simulink model "V5_Diagrama_completo_prolijo"  (R2023b)
settings: Solver=VariableStepAuto  StartTime=0.0  StopTime=15  FixedStep=0.00001  RelTol=1e-3
values from neighbouring files (symbols this model uses):
  A_corriente = [0 1; -wn_corriente^2 -2*zeta_corriente*wn_corriente]    [SensoresReales.m]
  A_inv = [0 1; -wn_inv^2 -2*zeta_inv*wn_inv]    [SensoresReales.m]
  A_temp = -1/tau_temp    (= -0.05)    [SensoresReales.m]
  A_tita = [0 1; -wn_tita^2 -2*zeta_tita*wn_tita]    [SensoresReales.m]
  B_corriente = [0; wn_corriente^2]    [SensoresReales.m]
  B_inv = [0; wn_inv^2]    [SensoresReales.m]
  B_temp = 1/tau_temp    (= 0.05)    [SensoresReales.m]
  B_tita = [0; wn_tita^2]    [SensoresReales.m]
  ba = Jeq * n * wn    [PolosPID.m]
  C_corriente = [1 0]    [SensoresReales.m]
  C_inv = [1 0]    [SensoresReales.m]
  C_temp = 1    [SensoresReales.m]
  C_tita = [1 0]    [SensoresReales.m]
  D_corriente = 0    [SensoresReales.m]
  D_inv = 0    [SensoresReales.m]
  D_temp = 0    [SensoresReales.m]
  D_tita = 0    [SensoresReales.m]
  ketita = double(sol.ketita_s)    [PIDPolosObsReducidoEst.m]    (also in PolosObsReducidoEst.m)
  kew = double(sol.kew_s)    [PIDPolosObsReducidoEst.m]    (also in PolosObsReducidoEst.m)
  kewint = double(sol.kewint_s)    [PIDPolosObsReducidoEst.m]    (also in PolosObsReducidoEst.m = 0)
  Ksa = Jeq * n * wn^2    [PolosPID.m]
  Ksia = Jeq * wn^3    [PolosPID.m]
  Ra_prima = Lq/Tau    [RaLazoControlCorriente.m]
  Vs_max = 48 * sqrt(2) / sqrt(3)    [SensoresReales.m]
undefined symbols (not defined in the file or in its folder): alfa, beq, Cts, g, id0, io0, iq0, Jeq, KEeq, kl, KTeq, lambda_m, Ld, Lls, Lq, Pp, r, Rs, Rts_amb, tita0, Ts0, wm0
libraries: simulink_extras x8, eeTransforms x4, SignalEditorBlockLib x3, simulink x3
settings Model: Creator=Julian  LastModifiedBy=Julian

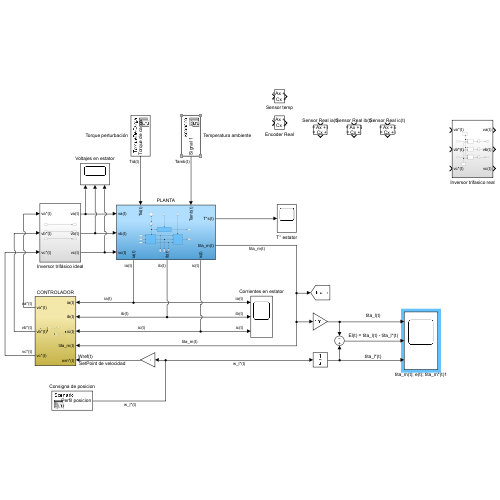
[thumbnail: Simulink's stored preview of the top-level diagram]
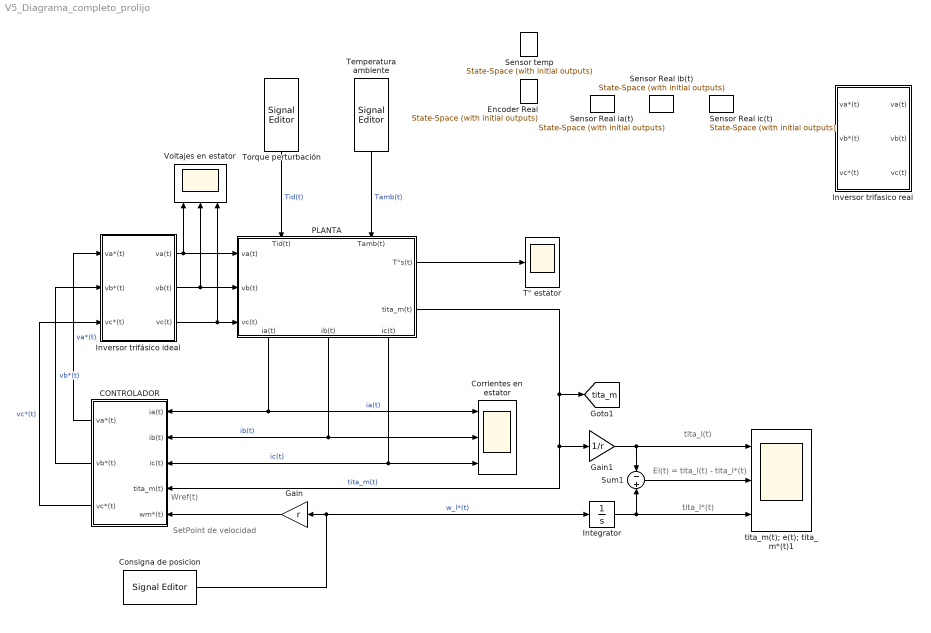
== system V5_Diagrama_completo_prolijo ==
  note: Wref(t)
  note: El(t) = tita_l(t) - tita_l*(t)
  note: tita_l*(t)
  note: tita_l(t)
  note: SetPoint de velocidad
  CONTROLADOR : Subsystem
  Consigna de posicion : SignalEditorBlockLib/Signal Editor  FileName=C:\Users\Julian\OneDrive\Documentos\UNC\Cuarto\AyME\Proyecto\Simulink\Señales\PerfilTrapezoidalVelocidadMejorado.mat  ActiveScenario=Scenario  ActiveSignal=Perfil posicion  IsBus=off  OutputBusObjectStr=Bus: BusObject  SampleTime=0  ZeroCross=off  OutputAfterFinalValue=Setting to zero  Unit=inherit  PreserveSignalName=on  ApplySigPropsToAllScenarios=on  ApplySigPropsToAllSignals=off
  Corrientes en estator : Scope  NumInputPorts=3
  Encoder Real : simulink_extras/Additional Linear/State-Space (with initial outputs)  A=A_tita  B=B_tita  C=C_tita  D=D_tita  U0=0  Y0=0
  Gain : Gain  Gain=r
  Gain1 : Gain  Gain=1/r
  Integrator : Integrator
  Inversor trifasico real : Subsystem
  Inversor trifásico ideal : Subsystem
  PLANTA : Subsystem
      settings: PortSchema="{\"entries\":[{\"content\":{\"sides\":[{\"content\":{\"connectorIds\":[\"In1\",\"In2\",\"In3\"]},\"type\":\"ConnectorPlacement.EquallySpacedRectSide\",\"uuid\":\"c9ff8e03-575d-49b6-9d53-263c6173ec7a\"},{\"content\":{\"connectorIds\":[\"Out1\",\"Out2\"],\"side\":\"RIGHT\"},\"type\":\"ConnectorPlacement.EquallySpacedRectSide\",\"uuid\":\"b812656a-111e-4032-91bd-eba1e3276cdf\"},{\"content\":{\"connectorIds\":[\"In4\",\"In5\"],\"side\":\"TOP\"},\"type\":\"ConnectorPlacement.EquallySpacedRectSide\",\"uuid\":\"1a03caaa-7f6e-4ad3-ab54-ee47607f786a\"},{\"content\":{\"connectorIds\":[\"Out3\",\"Out4\",\"Out5\"],\"side\":\"BOTTOM\"},\"type\":\"ConnectorPlacement.EquallySpacedRectSide\",\"uuid\":\"9d23a867-d392-4f38-a76b-2655c4618fc4\"}]},\"type\":\"ConnectorPlacement.EquallySpacedConnector\",\"uuid\":\"9323b1ce-1fa4-461e-b8aa-3e94b35b1dab\"}],\"packageUris\":[\"http://schema.mathworks.com/mf0/Connector/R2020b\"],\"version\":\"1.0\"}"
  Sensor Real ia(t) : simulink_extras/Additional Linear/State-Space (with initial outputs)  A=A_corriente  B=B_corriente  C=C_corriente  D=D_corriente  U0=0  Y0=0
  Sensor Real ib(t) : simulink_extras/Additional Linear/State-Space (with initial outputs)  A=A_corriente  B=B_corriente  C=C_corriente  D=D_corriente  U0=0  Y0=0
  Sensor Real ic(t) : simulink_extras/Additional Linear/State-Space (with initial outputs)  A=A_corriente  B=B_corriente  C=C_corriente  D=D_corriente  U0=0  Y0=0
  Sensor temp : simulink_extras/Additional Linear/State-Space (with initial outputs)  A=A_temp  B=B_temp  C=C_temp  D=D_temp  U0=40  Y0=40
  Sum1 : Sum  Inputs=-|+
  Temperatura ambiente : SignalEditorBlockLib/Signal Editor  FileName=C:\Users\Julian\OneDrive\Documentos\UNC\Cuarto\AyME\Proyecto\Simulink\Señales\Temperatura ambiente Tamb(t).mat  ActiveScenario=Scenario  ActiveSignal=Signal 1  IsBus=off  OutputBusObjectStr=Bus: BusObject  SampleTime=0  ZeroCross=off  OutputAfterFinalValue=Setting to zero  Unit=inherit  PreserveSignalName=on  ApplySigPropsToAllScenarios=on  ApplySigPropsToAllSignals=off
  Torque perturbación : SignalEditorBlockLib/Signal Editor  FileName=C:\Users\Julian\OneDrive\Documentos\UNC\Cuarto\AyME\Proyecto\Simulink\Señales\Torque de carga Tdl(t).mat  ActiveScenario=TorqueDeCarga  ActiveSignal=Torque de carga  IsBus=off  OutputBusObjectStr=Bus: BusObject  SampleTime=0  ZeroCross=off  OutputAfterFinalValue=Setting to zero  Unit=N*m  PreserveSignalName=on  ApplySigPropsToAllScenarios=on  ApplySigPropsToAllSignals=off
  T° estator : Scope
  Voltajes en estator : Scope  NumInputPorts=3
  tita_m(t); e(t); tita_m*(t)1 : Scope  NumInputPorts=3
  tag scope: tita_m=global
  wires:
  Gain/1 -> CONTROLADOR/5(wm*(t))
  Gain1/1 -> tita_m(t); e(t); tita_m*(t)1/1, Sum1/1
  Sum1/1 -> tita_m(t); e(t); tita_m*(t)1/2
  Integrator/1 -> Sum1/2, tita_m(t); e(t); tita_m*(t)1/3
  Temperatura ambiente/1 -> PLANTA/5(Tamb(t))  "Tamb(t)"
  Torque perturbación/1 -> PLANTA/4(Tid(t))  "Tid(t)"
  PLANTA/5(ic(t)) -> CONTROLADOR/3(ic(t)), Corrientes en estator/3  "ic(t)"
  PLANTA/4(ib(t)) -> CONTROLADOR/2(ib(t)), Corrientes en estator/2  "ib(t)"
  PLANTA/3(ia(t)) -> CONTROLADOR/1(ia(t)), Corrientes en estator/1  "ia(t)"
  PLANTA/2(tita_m(t)) -> CONTROLADOR/4(tita_m(t)), Gain1/1, [tita_m]  "tita_m(t)"
  CONTROLADOR/1(va*(t)) -> Inversor trifásico ideal/1(va*(t))  "va*(t)"
  CONTROLADOR/2(vb*(t)) -> Inversor trifásico ideal/2(vb*(t))  "vb*(t)"
  CONTROLADOR/3(vc*(t)) -> Inversor trifásico ideal/3(vc*(t))  "vc*(t)"
  Inversor trifásico ideal/1(va(t)) -> PLANTA/1(va(t)), Voltajes en estator/1
  Inversor trifásico ideal/2(vb(t)) -> PLANTA/2(vb(t)), Voltajes en estator/2
  Inversor trifásico ideal/3(vc(t)) -> Voltajes en estator/3, PLANTA/3(vc(t))
  Consigna de posicion/1 -> Integrator/1, Gain/1  "w_l*(t)"
  PLANTA/1(T°s(t)) -> T° estator/1

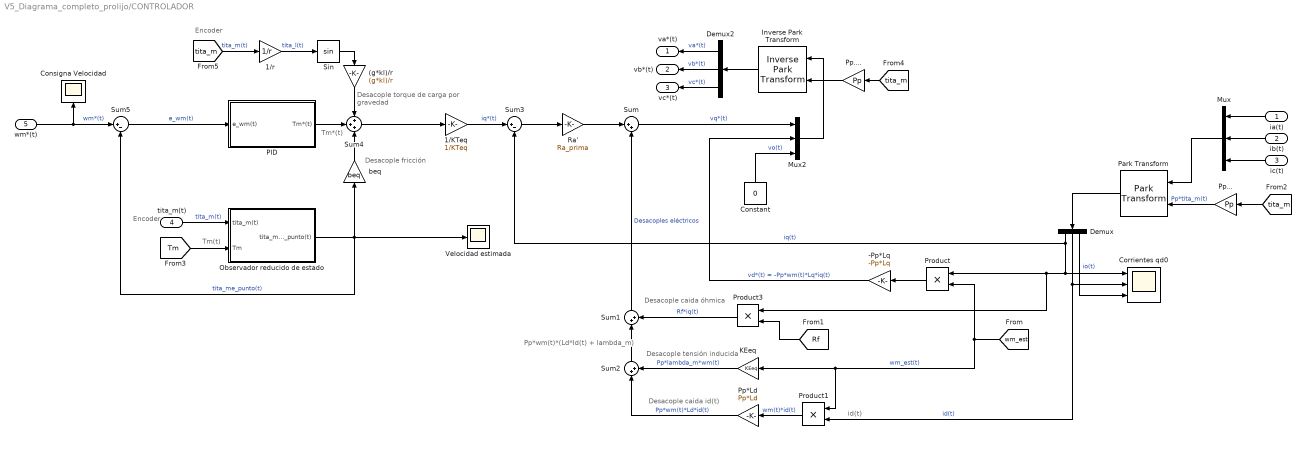
== system V5_Diagrama_completo_prolijo/CONTROLADOR ==
  note: id(t)
  note: Desacople caida id(t)
  note: Encoder
  note: Desacople caida óhmica
  note: Desacople fricción
  note: Tm(t)
  note: Tm*(t)
  note: Desacople tensión inducida
  note: Pp*wm(t)*(Ld*Id(t) + lambda_m)
  note: Encoder
  note: Desacople torque
      | de carga por gravedad
  ia(t) : Inport
  ib(t) : Inport  Port=2
  ic(t) : Inport  Port=3
  tita_m(t) : Inport  Port=4
  wm*(t) : Inport  Port=5
  (g*kl)/r : Gain  Gain=(g*kl)/r
  -Pp*Lq : Gain  Gain=-Pp*Lq
  1/KTeq : Gain  Gain=1/KTeq
  1/r : Gain  Gain=1/r
  Consigna Velocidad : Scope
  Constant : Constant  Value=0
  Corrientes qd0 : Scope  NumInputPorts=3
  Demux : Demux  Outputs=3
  Demux2 : Demux  Outputs=3
  Inverse Park Transform : eeTransforms/Inverse Park Transform  AxisAlignment=Q-axis  PowerInvariant=off
      settings: LibrarySourceBlock=|
      | ee_sl_lib/Mathematical
      | Transforms/Inverse
      | Park Transform
  KEeq : Gain  Gain=KEeq
  Mux : Mux  Inputs=3
  Mux2 : Mux  Inputs=3
  Observador reducido de estado : Subsystem
  PID : Subsystem
  Park Transform : eeTransforms/Park Transform  AxisAlignment=Q-axis  PowerInvariant=off
      settings: LibrarySourceBlock=|
      | ee_sl_lib/Mathematical
      | Transforms/Park Transform
  Pp*Ld : Gain  Gain=Pp*Ld
  Pp... : Gain  Gain=Pp
  Pp.... : Gain  Gain=Pp
  Product : Product
  Product1 : Product
  Product3 : Product
  Ra' : Gain  Gain=Ra_prima
  Sin : Trigonometry
  Sum : Sum  Inputs=|++
  Sum1 : Sum  Inputs=|++
  Sum2 : Sum  Inputs=|++
  Sum3 : Sum  Inputs=|+-
  Sum4 : Sum  Inputs=+++
  Sum5 : Sum  Inputs=|+-
  Velocidad estimada : Scope
  beq : Gain  Gain=beq
  va*(t) : Outport
  vb*(t) : Outport  Port=2
  vc*(t) : Outport  Port=3
  wires:
  Mux/1 -> Park Transform/1
  [wm_est] -> Product1/1, KEeq/1, Product/2  "wm_est(t)"
  [tita_m] -> Pp..../1
  Pp..../1 -> Inverse Park Transform/2
  Demux2/2 -> vb*(t)/1  "vb*(t)"
  Sum3/1 -> Ra'/1
  Constant/1 -> Mux2/3  "vo(t)"
  Demux2/1 -> va*(t)/1  "va*(t)"
  -Pp*Lq/1 -> Mux2/2  "vd*(t) = -Pp*wm(t)*Lq*iq(t)"
  Product3/1 -> Sum1/2  "Rf*iq(t)"
  [tita_m] -> Pp.../1
  Ra'/1 -> Sum/1
  Inverse Park Transform/1 -> Demux2/1
  KEeq/1 -> Sum2/2  "Pp*lambda_m*wm(t)"
  Product1/1 -> Pp*Ld/1  "wm(t)*id(t)"
  Mux2/1 -> Inverse Park Transform/1
  Sum2/1 -> Sum1/1
  wm*(t)/1 -> Sum5/1, Consigna Velocidad/1  "wm*(t)"
  Pp*Ld/1 -> Sum2/1  "Pp*wm(t)*Ld*id(t)"
  1/KTeq/1 -> Sum3/1  "iq*(t)"
  Product/1 -> -Pp*Lq/1
  ia(t)/1 -> Mux/1
  Park Transform/1 -> Demux/1
  Pp.../1 -> Park Transform/2  "Pp*tita_m(t)"
  Sum/1 -> Mux2/1  "vq*(t)"
  Demux2/3 -> vc*(t)/1  "vc*(t)"
  ib(t)/1 -> Mux/2
  tita_m(t)/1 -> Observador reducido de estado/1(tita_m(t))  "tita_m(t)"
  [Tm] -> Observador reducido de estado/2(Tm)
  [Rf] -> Product3/2
  ic(t)/1 -> Mux/3
  Sum5/1 -> PID/1(e_wm(t))  "e_wm(t)"
  Sum1/1 -> Sum/2  "Desacoples eléctricos"
  PID/1(Tm*(t)) -> Sum4/2
  Sum4/1 -> 1/KTeq/1
  beq/1 -> Sum4/3
  Observador reducido de estado/1(tita_me_punto(t)) -> beq/1, Velocidad estimada/1, Sum5/2  "tita_me_punto(t)"
  Demux/3 -> Corrientes qd0/3  "io(t)"
  Demux/2 -> Product1/2, Corrientes qd0/2  "id(t)"
  Demux/1 -> Sum3/2, Corrientes qd0/1, Product/1, Product3/1  "iq(t)"
  1/r/1 -> Sin/1  "tita_l(t)"
  Sin/1 -> (g*kl)/r/1
  [tita_m] -> 1/r/1  "tita_m(t)"
  (g*kl)/r/1 -> Sum4/1

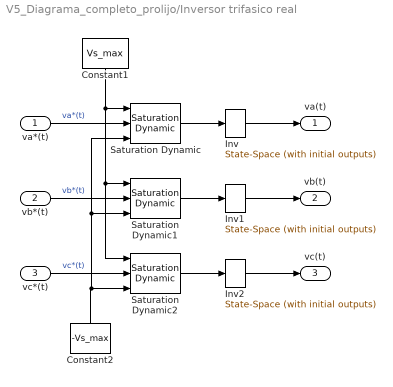
== system V5_Diagrama_completo_prolijo/Inversor trifasico real ==
  va*(t) : Inport
  vb*(t) : Inport  Port=2
  vc*(t) : Inport  Port=3
  Constant1 : Constant  Value=Vs_max
  Constant2 : Constant  Value=-Vs_max
  Inv : simulink_extras/Additional Linear/State-Space (with initial outputs)  A=A_inv  B=B_inv  C=C_inv  D=D_inv  U0=0  Y0=0
  Inv1 : simulink_extras/Additional Linear/State-Space (with initial outputs)  A=A_inv  B=B_inv  C=C_inv  D=D_inv  U0=0  Y0=0
  Inv2 : simulink_extras/Additional Linear/State-Space (with initial outputs)  A=A_inv  B=B_inv  C=C_inv  D=D_inv  U0=0  Y0=0
  Saturation Dynamic : simulink/Discontinuities/Saturation Dynamic  OutMin=[]  OutMax=[]  OutDataTypeStr=Inherit: Same as second input  OutDataType=fixdt(1, 16)  OutScaling=2^-10  DoSatur=off
  Saturation Dynamic1 : simulink/Discontinuities/Saturation Dynamic  OutMin=[]  OutMax=[]  OutDataTypeStr=Inherit: Same as second input  OutDataType=fixdt(1, 16)  OutScaling=2^-10  DoSatur=off
  Saturation Dynamic2 : simulink/Discontinuities/Saturation Dynamic  OutMin=[]  OutMax=[]  OutDataTypeStr=Inherit: Same as second input  OutDataType=fixdt(1, 16)  OutScaling=2^-10  DoSatur=off
  va(t) : Outport
  vb(t) : Outport  Port=2
  vc(t) : Outport  Port=3
  wires:
  Inv/1 -> va(t)/1
  Constant2/1 -> Saturation Dynamic2/3, Saturation Dynamic/3, Saturation Dynamic1/3
  va*(t)/1 -> Saturation Dynamic/2  "va*(t)"
  Saturation Dynamic2/1 -> Inv2/1
  vc*(t)/1 -> Saturation Dynamic2/2  "vc*(t)"
  vb*(t)/1 -> Saturation Dynamic1/2  "vb*(t)"
  Saturation Dynamic1/1 -> Inv1/1
  Saturation Dynamic/1 -> Inv/1
  Constant1/1 -> Saturation Dynamic2/1, Saturation Dynamic1/1, Saturation Dynamic/1
  Inv2/1 -> vc(t)/1
  Inv1/1 -> vb(t)/1

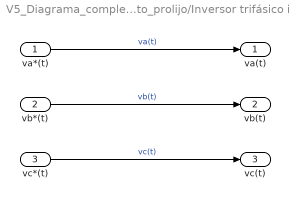
== system V5_Diagrama_completo_prolijo/Inversor trifásico ideal ==
  va*(t) : Inport
  vb*(t) : Inport  Port=2
  vc*(t) : Inport  Port=3
  va(t) : Outport
  vb(t) : Outport  Port=2
  vc(t) : Outport  Port=3
  wires:
  vc*(t)/1 -> vc(t)/1  "vc(t)"
  va*(t)/1 -> va(t)/1  "va(t)"
  vb*(t)/1 -> vb(t)/1  "vb(t)"

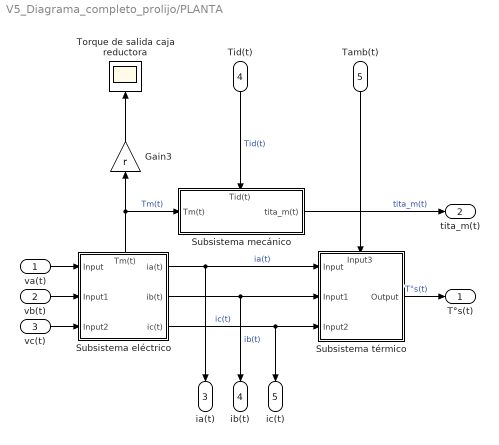
== system V5_Diagrama_completo_prolijo/PLANTA ==
  va(t) : Inport
  vb(t) : Inport  Port=2
  vc(t) : Inport  Port=3
  Tid(t) : Inport  Port=4
  Tamb(t) : Inport  Port=5
  Gain3 : Gain  Gain=r
  Subsistema eléctrico : Subsystem
      settings: PortSchema="{\"entries\":[{\"content\":{\"sides\":[{\"content\":{\"connectorIds\":[\"In1\",\"In2\",\"In3\"]},\"type\":\"ConnectorPlacement.EquallySpacedRectSide\",\"uuid\":\"55314de5-b6ab-4161-b15d-819ac9b3d610\"},{\"content\":{\"connectorIds\":[\"Out1\",\"Out2\",\"Out3\"],\"side\":\"RIGHT\"},\"type\":\"ConnectorPlacement.EquallySpacedRectSide\",\"uuid\":\"6d89c228-26ff-4db5-b942-5bfef0be2fde\"},{\"content\":{\"connectorIds\":[\"Out4\"],\"side\":\"TOP\"},\"type\":\"ConnectorPlacement.EquallySpacedRectSide\",\"uuid\":\"a52f3ca3-a7f6-4886-b92b-9c9e6a107711\"}]},\"type\":\"ConnectorPlacement.EquallySpacedConnector\",\"uuid\":\"22991da4-d60d-4ddc-8bfe-b68e23663f11\"}],\"packageUris\":[\"http://schema.mathworks.com/mf0/Connector/R2020b\"],\"version\":\"1.0\"}"
  Subsistema mecánico : Subsystem
      settings: PortSchema="{\"entries\":[{\"content\":{\"sides\":[{\"content\":{\"connectorIds\":[\"In1\"]},\"type\":\"ConnectorPlacement.EquallySpacedRectSide\",\"uuid\":\"db0c31ff-fb9a-4cce-bd75-6b297d65744d\"},{\"content\":{\"connectorIds\":[\"Out1\"],\"side\":\"RIGHT\"},\"type\":\"ConnectorPlacement.EquallySpacedRectSide\",\"uuid\":\"ab44173d-bb84-4ea2-b7b7-ef15b1ff9d5e\"},{\"content\":{\"connectorIds\":[\"In2\"],\"side\":\"TOP\"},\"type\":\"ConnectorPlacement.EquallySpacedRectSide\",\"uuid\":\"a2ba5669-abba-4e87-b14b-37ec0d904023\"}]},\"type\":\"ConnectorPlacement.EquallySpacedConnector\",\"uuid\":\"7722c9ef-afaa-4930-9e2a-97c0dfb446ab\"}],\"packageUris\":[\"http://schema.mathworks.com/mf0/Connector/R2020b\"],\"version\":\"1.0\"}"
  Subsistema térmico : Subsystem
      settings: PortSchema="{\"entries\":[{\"content\":{\"sides\":[{\"content\":{\"connectorIds\":[\"In1\",\"In2\",\"In3\"]},\"type\":\"ConnectorPlacement.EquallySpacedRectSide\",\"uuid\":\"499bb5e3-da94-498d-be5e-1974ba0b4a58\"},{\"content\":{\"connectorIds\":[\"Out1\"],\"side\":\"RIGHT\"},\"type\":\"ConnectorPlacement.EquallySpacedRectSide\",\"uuid\":\"13ea5dea-e51e-4770-b579-88e3e6e50884\"},{\"content\":{\"connectorIds\":[\"In4\"],\"side\":\"TOP\"},\"type\":\"ConnectorPlacement.EquallySpacedRectSide\",\"uuid\":\"72517ed1-a98f-428e-86e2-c370e237c602\"}]},\"type\":\"ConnectorPlacement.EquallySpacedConnector\",\"uuid\":\"7e0eda24-12d6-49d0-ad1f-024c88e78140\"}],\"packageUris\":[\"http://schema.mathworks.com/mf0/Connector/R2020b\"],\"version\":\"1.0\"}"
  Torque de salida caja reductora : Scope
  T°s(t) : Outport
  tita_m(t) : Outport  Port=2
  ia(t) : Outport  Port=3
  ib(t) : Outport  Port=4
  ic(t) : Outport  Port=5
  wires:
  Tamb(t)/1 -> Subsistema térmico/4(Input3)
  Subsistema eléctrico/3(ic(t)) -> Subsistema térmico/3(Input2), ic(t)/1  "ic(t)"
  Subsistema eléctrico/1(ia(t)) -> Subsistema térmico/1(Input), ia(t)/1  "ia(t)"
  Subsistema térmico/1(Output) -> T°s(t)/1  "T°s(t)"
  Subsistema eléctrico/4(Tm(t)) -> Gain3/1, Subsistema mecánico/1(Tm(t))  "Tm(t)"
  Subsistema eléctrico/2(ib(t)) -> Subsistema térmico/2(Input1), ib(t)/1  "ib(t)"
  Subsistema mecánico/1(tita_m(t)) -> tita_m(t)/1  "tita_m(t)"
  va(t)/1 -> Subsistema eléctrico/1(Input)
  vb(t)/1 -> Subsistema eléctrico/2(Input1)
  Tid(t)/1 -> Subsistema mecánico/2(Tid(t))  "Tid(t)"
  vc(t)/1 -> Subsistema eléctrico/3(Input2)
  Gain3/1 -> Torque de salida caja reductora/1

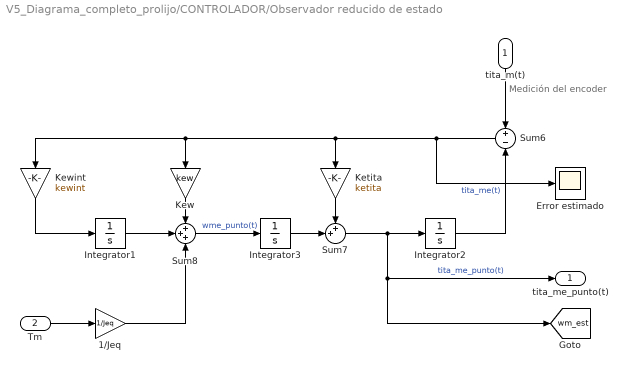
== system V5_Diagrama_completo_prolijo/CONTROLADOR/Observador reducido de estado ==
  note: Medición del encoder
  tita_m(t) : Inport
  Tm : Inport  Port=2
  1/Jeq : Gain  Gain=1/Jeq
  Error estimado : Scope
  Integrator1 : Integrator
  Integrator2 : Integrator
  Integrator3 : Integrator
  Ketita : Gain  Gain=ketita
  Kew : Gain  Gain=kew
  Kewint : Gain  Gain=kewint
  Sum6 : Sum  Inputs=+-
  Sum7 : Sum  Inputs=++|
  Sum8 : Sum  Inputs=+++
  tita_me_punto(t) : Outport
  tag scope: wm_est=global
  wires:
  Sum7/1 -> [wm_est], tita_me_punto(t)/1, Integrator2/1  "tita_me_punto(t)"
  Sum6/1 -> Error estimado/1, Kewint/1, Kew/1, Ketita/1
  Integrator3/1 -> Sum7/2
  Integrator2/1 -> Sum6/2  "tita_me(t)"
  Kew/1 -> Sum8/1
  Ketita/1 -> Sum7/1
  Sum8/1 -> Integrator3/1  "wme_punto(t)"
  tita_m(t)/1 -> Sum6/1
  Tm/1 -> 1/Jeq/1
  1/Jeq/1 -> Sum8/3
  Kewint/1 -> Integrator1/1
  Integrator1/1 -> Sum8/2

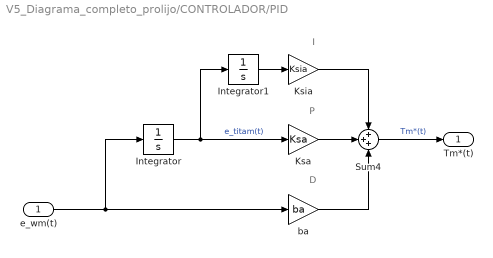
== system V5_Diagrama_completo_prolijo/CONTROLADOR/PID ==
  note: D
  note: I
  note: P
  e_wm(t) : Inport
  Integrator : Integrator
  Integrator1 : Integrator
  Ksa : Gain  Gain=Ksa
  Ksia : Gain  Gain=Ksia
  Sum4 : Sum  Inputs=+++
  ba : Gain  Gain=ba
  Tm*(t) : Outport
  wires:
  Integrator1/1 -> Ksia/1
  e_wm(t)/1 -> Integrator/1, ba/1
  ba/1 -> Sum4/3
  Sum4/1 -> Tm*(t)/1  "Tm*(t)"
  Integrator/1 -> Integrator1/1, Ksa/1  "e_titam(t)"
  Ksia/1 -> Sum4/1
  Ksa/1 -> Sum4/2

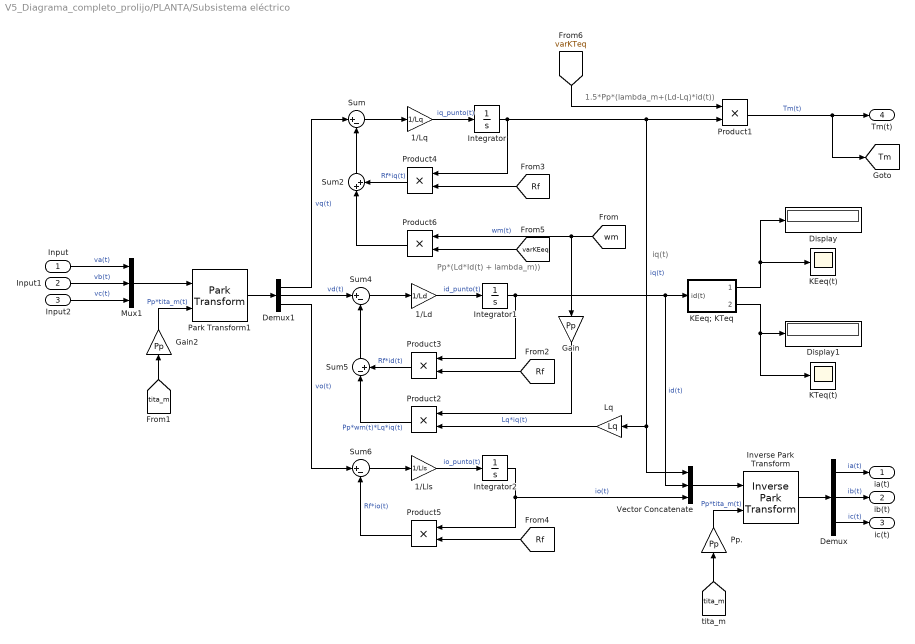
== system V5_Diagrama_completo_prolijo/PLANTA/Subsistema eléctrico ==
  note: 1.5*Pp*(lambda_m+(Ld-Lq)*id(t))
  note: iq(t)
  note: Pp*(Ld*Id(t) + lambda_m))
  Input : Inport
  Input1 : Inport  Port=2
  Input2 : Inport  Port=3
  1/Ld : Gain  Gain=1/Ld
  1/Lls : Gain  Gain=1/Lls
  1/Lq : Gain  Gain=1/Lq
  Demux : Demux  Outputs=3
  Demux1 : Demux  Outputs=3
  Display : Display
  Display1 : Display
  Gain : Gain  Gain=Pp
  Gain2 : Gain  Gain=Pp
  Integrator : Integrator  InitialCondition=iq0
  Integrator1 : Integrator  InitialCondition=id0
  Integrator2 : Integrator  InitialCondition=io0
  Inverse Park Transform : eeTransforms/Inverse Park Transform  AxisAlignment=Q-axis  PowerInvariant=off
      settings: LibrarySourceBlock=|
      | ee_sl_lib/Mathematical
      | Transforms/Inverse
      | Park Transform
  KEeq(t) : Scope
  KEeq; KTeq : Subsystem
  KTeq(t) : Scope
  Lq : Gain  Gain=Lq
  Mux1 : Mux  Inputs=3
  Park Transform1 : eeTransforms/Park Transform  AxisAlignment=Q-axis  PowerInvariant=off
      settings: LibrarySourceBlock=|
      | ee_sl_lib/Mathematical
      | Transforms/Park Transform
  Pp. : Gain  Gain=Pp
  Product{1..6} (6 alike) : Product
  Sum : Sum  Inputs=|+-
  Sum2 : Sum  Inputs=|++
  Sum4 : Sum  Inputs=|+-
  Sum5 : Sum  Inputs=|-+
  Sum6 : Sum  Inputs=|+-
  Vector Concatenate : Concatenate  NumInputs=3
  ia(t) : Outport
  ib(t) : Outport  Port=2
  ic(t) : Outport  Port=3
  Tm(t) : Outport  Port=4
  tag scope: Tm=global
  wires:
  Sum4/1 -> 1/Ld/1
  Demux1/1 -> Sum/1  "vq(t)"
  Integrator/1 -> Product4/1, Product1/2, Lq/1, Vector Concatenate/1  "iq(t)"
  Product4/1 -> Sum2/2  "Rf*iq(t)"
  Pp./1 -> Inverse Park Transform/2  "Pp*tita_m(t)"
  Lq/1 -> Product2/2  "Lq*iq(t)"
  Sum/1 -> 1/Lq/1
  Sum2/1 -> Sum/2
  Demux1/3 -> Sum6/1  "vo(t)"
  Vector Concatenate/1 -> Inverse Park Transform/1
  1/Ld/1 -> Integrator1/1  "id_punto(t)"
  Inverse Park Transform/1 -> Demux/1
  1/Lls/1 -> Integrator2/1  "io_punto(t)"
  Sum5/1 -> Sum4/2
  Demux/3 -> ic(t)/1  "ic(t)"
  Demux/1 -> ia(t)/1  "ia(t)"
  Product3/1 -> Sum5/2  "Rf*id(t)"
  Demux/2 -> ib(t)/1  "ib(t)"
  Integrator2/1 -> Product5/1, Vector Concatenate/3  "io(t)"
  [tita_m] -> Pp./1
  Demux1/2 -> Sum4/1  "vd(t)"
  Product6/1 -> Sum2/1
  Product5/1 -> Sum6/2  "Rf*io(t)"
  Product2/1 -> Sum5/1  "Pp*wm(t)*Lq*iq(t)"
  1/Lq/1 -> Integrator/1  "iq_punto(t)"
  Sum6/1 -> 1/Lls/1
  [wm] -> Product6/1, Gain/1  "wm(t)"
  Product1/1 -> Tm(t)/1, [Tm]  "Tm(t)"
  Input1/1 -> Mux1/2  "vb(t)"
  Gain2/1 -> Park Transform1/2  "Pp*tita_m(t)"
  Input2/1 -> Mux1/3  "vc(t)"
  Mux1/1 -> Park Transform1/1
  Input/1 -> Mux1/1  "va(t)"
  [tita_m] -> Gain2/1
  Park Transform1/1 -> Demux1/1
  [Rf] -> Product3/2
  [Rf] -> Product4/2
  [Rf] -> Product5/2
  Integrator1/1 -> Product3/1, Vector Concatenate/2, KEeq; KTeq/1(id(t))  "id(t)"
  KEeq; KTeq/2(KTeq(t)) -> KTeq(t)/1, Display1/1
  KEeq; KTeq/1(KEeq(t)) -> KEeq(t)/1, Display/1
  [varKEeq] -> Product6/2
  Gain/1 -> Product2/1
  [varKTeq] -> Product1/1

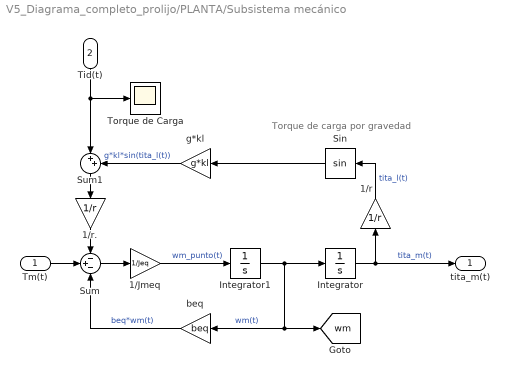
== system V5_Diagrama_completo_prolijo/PLANTA/Subsistema mecánico ==
  note: Torque de carga por gravedad
  Tm(t) : Inport
  Tid(t) : Inport  Port=2
  1/Jmeq : Gain  Gain=1/Jeq
  1/r : Gain  Gain=1/r
  1/r. : Gain  Gain=1/r
  Integrator : Integrator  InitialCondition=tita0
  Integrator1 : Integrator  InitialCondition=wm0
  Sin : Trigonometry
  Sum : Sum  Inputs=-+-
  Sum1 : Sum  Inputs=|++
  Torque de Carga : Scope
  beq : Gain  Gain=beq
  g*kl : Gain  Gain=g*kl
  tita_m(t) : Outport
  tag scope: wm=global
  wires:
  Integrator/1 -> tita_m(t)/1, 1/r/1  "tita_m(t)"
  1/r./1 -> Sum/1
  Integrator1/1 -> beq/1, [wm], Integrator/1  "wm(t)"
  1/r/1 -> Sin/1  "tita_l(t)"
  Sin/1 -> g*kl/1
  Sum/1 -> 1/Jmeq/1
  1/Jmeq/1 -> Integrator1/1  "wm_punto(t)"
  beq/1 -> Sum/3  "beq*wm(t)"
  Tm(t)/1 -> Sum/2
  Tid(t)/1 -> Sum1/1, Torque de Carga/1
  Sum1/1 -> 1/r./1
  g*kl/1 -> Sum1/2  "g*kl*sin(tita_l(t))"

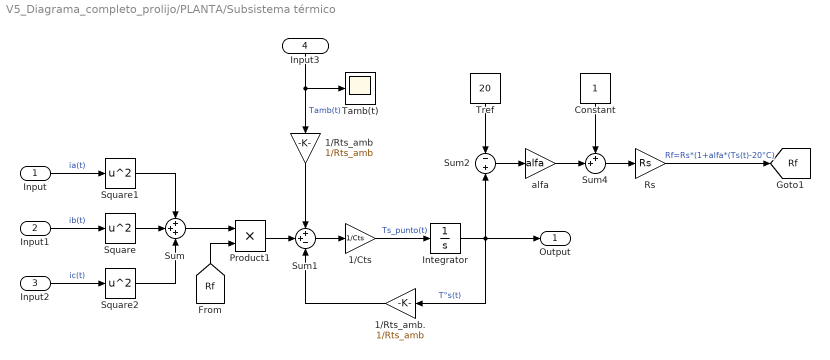
== system V5_Diagrama_completo_prolijo/PLANTA/Subsistema térmico ==
  Input : Inport
  Input1 : Inport  Port=2
  Input2 : Inport  Port=3
  Input3 : Inport  Port=4
  1/Cts : Gain  Gain=1/Cts
  1/Rts_amb : Gain  Gain=1/Rts_amb
  1/Rts_amb. : Gain  Gain=1/Rts_amb
  Constant : Constant
  Integrator : Integrator  InitialCondition=Ts0
  Product1 : Product
  Rs : Gain  Gain=Rs
  Square : Math  Operator=square
  Square1 : Math  Operator=square
  Square2 : Math  Operator=square
  Sum : Sum  Inputs=+++
  Sum1 : Sum  Inputs=++-
  Sum2 : Sum  Inputs=-+
  Sum4 : Sum  Inputs=++|
  Tamb(t) : Scope
  Tref : Constant  Value=20
  alfa : Gain  Gain=alfa
  Output : Outport
  tag scope: Rf=global
  wires:
  1/Rts_amb/1 -> Sum1/1
  Sum1/1 -> 1/Cts/1
  Product1/1 -> Sum1/2
  Sum/1 -> Product1/1
  Integrator/1 -> Sum2/2, Output/1, 1/Rts_amb./1  "T°s(t)"
  1/Cts/1 -> Integrator/1  "Ts_punto(t)"
  1/Rts_amb./1 -> Sum1/3
  Square/1 -> Sum/2
  Square1/1 -> Sum/1
  Square2/1 -> Sum/3
  Input/1 -> Square1/1  "ia(t)"
  Input1/1 -> Square/1  "ib(t)"
  Input2/1 -> Square2/1  "ic(t)"
  Sum2/1 -> alfa/1
  Constant/1 -> Sum4/1
  alfa/1 -> Sum4/2
  Rs/1 -> [Rf]  "Rf=Rs*(1+alfa*(Ts(t)-20°C)"
  [Rf] -> Product1/2
  Tref/1 -> Sum2/1
  Sum4/1 -> Rs/1
  Input3/1 -> 1/Rts_amb/1, Tamb(t)/1  "Tamb(t)"

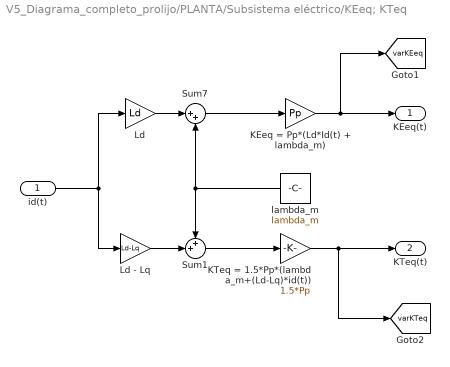
== system V5_Diagrama_completo_prolijo/PLANTA/Subsistema eléctrico/KEeq; KTeq ==
  id(t) : Inport
  "KEeq = Pp*(Ld*Id(t) + lambda_m) " : Gain  Gain=Pp
  "KTeq = 1.5*Pp*(lambda_m+(Ld-Lq)*id(t)) " : Gain  Gain=1.5*Pp
  Ld : Gain  Gain=Ld
  Ld - Lq : Gain  Gain=Ld-Lq
  Sum1 : Sum  Inputs=++|
  Sum7 : Sum  Inputs=|++
  lambda_m : Constant  Value=lambda_m
  KEeq(t) : Outport
  KTeq(t) : Outport  Port=2
  tag scope: varKEeq=global, varKTeq=global
  wires:
  Ld/1 -> Sum7/1
  Sum7/1 -> "KEeq = Pp*(Ld*Id(t) + lambda_m) "/1
  "KTeq = 1.5*Pp*(lambda_m+(Ld-Lq)*id(t)) "/1 -> KTeq(t)/1, [varKTeq]
  Sum1/1 -> "KTeq = 1.5*Pp*(lambda_m+(Ld-Lq)*id(t)) "/1
  id(t)/1 -> Ld/1, Ld - Lq/1
  Ld - Lq/1 -> Sum1/2
  lambda_m/1 -> Sum1/1, Sum7/2
  "KEeq = Pp*(Ld*Id(t) + lambda_m) "/1 -> [varKEeq], KEeq(t)/1
